simulink model "sampleModel2082"  (R2023a)
settings: Solver=VariableStepAuto  StartTime=0.0  StopTime=10.0  RelTol=1e-3
libraries: simulink x3, hdlsllib x2
settings Model: Creator=user1  LastModifiedBy=user1

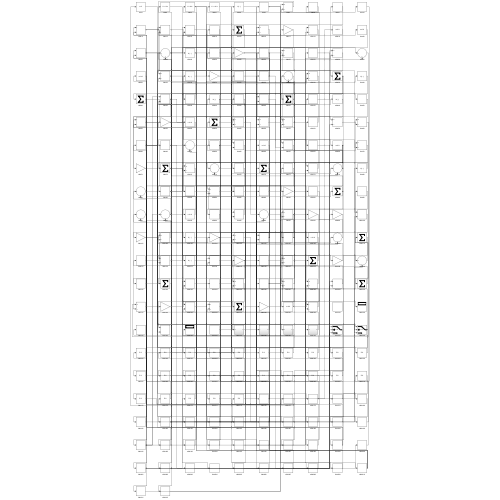
[thumbnail: Simulink's stored preview of the top-level diagram]
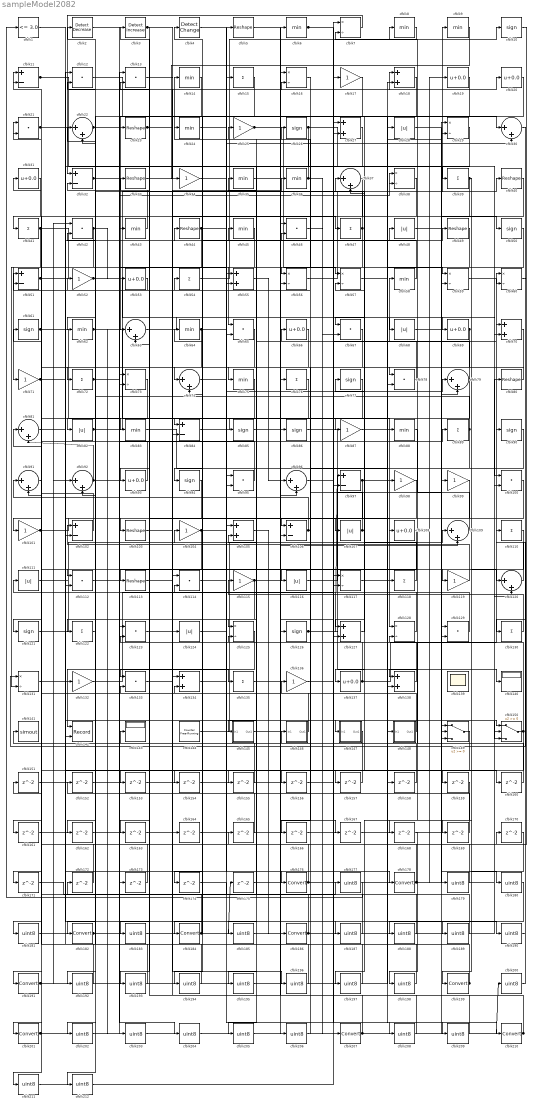
== system sampleModel2082 ==
  cfblk1 : hdlsllib/Logic and Bit Operations/Compare To Constant  relop=<=  const=3.0  OutDataTypeStr=boolean
  cfblk{10,26,50,61,77,85..86,90,94,121,126} (11 alike) : Signum
  cfblk{12..13,21,42,46,65,67,78,95,100,112,114,123,129,133} (15 alike) : DotProduct  OutDataTypeStr=Inherit: Inherit via internal rule
  cfblk{17,25,34,52,71,87,98..99,101,104,115,119,132,136} (14 alike) : Gain
  cfblk{11,32,51,84,97,102,106} (7 alike) : Sum  Inputs=+-
  cfblk{5,23,33,40,44,49,80,103,113} (9 alike) : Reshape
  cfblk{18,27,55,70,105,127,134,138} (8 alike) : Sum
  cfblk{28,48,68,82,107,111,116,124} (8 alike) : Abs  SaturateOnIntegerOverflow=off
  cfblk{19..20,31,53,66,69,93,108,137} (9 alike) : Bias  Bias=0.0  SaturateOnIntegerOverflow=off
  cfblk{22,30,37,63,74,79,81,91..92,96,109,120} (12 alike) : Sum  Inputs=|++
  cfblk{15,39,41,47,54,72,76,89,110,118,122,130,135} (13 alike) : Sum  Inputs=+
  cfblk{7,16,29,38,56..57,59..60,73,117,125,128,131} (13 alike) : Product  Inputs=*/  RndMeth=Zero  SaturateOnIntegerOverflow=on
  cfblk139 : Scope
      settings: Floating=on
  cfblk{6,8..9,14,24,35..36,43,45,58,62,64,75,83,88} (15 alike) : MinMax
  cfblk140 : Display
  cfblk141 : ToWorkspace  VariableName=simout  SaveFormat=Timeseries  SampleTime=-1
  cfblk142 : Record  FileSettingsInternal="{\"entries\":[{\"content\":{\"excelSettings\":{\"content\":{},\"type\":\"Streamout.ExcelSettings\"}},\"type\":\"Streamout.FileSettingStorage\",\"uuid\":\"\"}],\"packageUris\":[\"http:\\/\\/schema.mathworks.com\\/mf0\\/streamout_blocks\\/R2020a\"],\"version\":\"1.0\"}"  Layout=[1 1]  SignalsInternal="{\"entries\":[{\"content\":{\"signals\":[{\"content\":{\"blockPath\":[],\"dimensions\":[1],\"domain\":\"\",\"lineColor\":\"#a2142f\",\"plots\":[1],\"port\":1,\"signalID\":6656,\"signalName\":\"XY Graph:1\"},\"type\":\"RecordBlkView.Signal\",\"uuid\":\"\"},{\"content\":{\"blockPath\":[],\"dimensions\":[1],\"domain\":\"\",\"lineColor\":\"#139fff\",\"plots\":[1],\"port\":2,\"signalID\":6659,\"signalName\":\"XY Graph:2\"},\"type\":\"RecordBlkView.Signal\",\"uuid\":\"\"}]},\"type\":\"RecordBlkView.InputSignals\",\"uuid\":\"\"}],\"packageUris\":[\"http:\\/\\/schema.mathworks.com\\/mf0\\/streamout_blocks\\/R2020a\"],\"version\":\"1.0\"}"  VisualizationBindings="{\"xyplotplugin\":{\"info\":[{\"series\":[{\"bindingParametersList\":[{\"parameter\":\"X-Axis\",\"signalID\":6656,\"signalName\":\"XY Graph:1\"},{\"parameter\":\"Y-Axis\",\"signalID\":6659,\"signalName\":\"XY Graph:2\"}],\"seriesID\":13052}],\"subplotID\":1}]}}"  CompatibilityTag=XY  st=-1
  cfblk143 : Display
  cfblk144 : hdlsllib/Sources/Counter Free-Running  NumBits=16  tsamp=-1
  cfblk145 : Subsystem
      settings: LibrarySourceBlock=|
      | hdlsllib/Ports &
      | Subsystems/Subsystem
  cfblk146 : Subsystem
      settings: LibrarySourceBlock=|
      | hdlsllib/Ports &
      | Subsystems/Subsystem
  cfblk147 : Subsystem
      settings: LibrarySourceBlock=|
      | hdlsllib/Ports &
      | Subsystems/Subsystem
  cfblk148 : Subsystem
      settings: LibrarySourceBlock=|
      | hdlsllib/Ports &
      | Subsystems/Subsystem
  cfblk149 : Switch  SaturateOnIntegerOverflow=off  InputSameDT=off
  cfblk150 : Switch  SaturateOnIntegerOverflow=off  InputSameDT=off
  cfblk{151..175} (25 alike) : Delay  SampleTime=1
  cfblk{176,178,182,184,186,191,199,201,207,210} (10 alike) : DataTypeConversion  SaturateOnIntegerOverflow=off  RndMeth=Floor
  cfblk{177,179..181,183,185,187..190,192..198,200,202..206,208..209,211..212} (27 alike) : DataTypeConversion  OutDataTypeStr=uint8  SaturateOnIntegerOverflow=off  RndMeth=Floor
  cfblk2 : simulink/Logic and Bit Operations/Detect Decrease  vinit=0.0  OutDataTypeStr=boolean
      settings: LibrarySourceBlock=|
      | hdlsllib/Logic and Bit
      | Operations/Detect
      | Decrease
  cfblk3 : simulink/Logic and Bit Operations/Detect Increase  vinit=0.0  OutDataTypeStr=boolean
      settings: LibrarySourceBlock=|
      | hdlsllib/Logic and Bit
      | Operations/Detect
      | Increase
  cfblk4 : simulink/Logic and Bit Operations/Detect Change  vinit=0  OutDataTypeStr=boolean
      settings: LibrarySourceBlock=|
      | hdlsllib/Logic and Bit
      | Operations/Detect
      | Change
  wires:
  cfblk79/1 -> cfblk58/1, cfblk37/2, cfblk171/1
  cfblk101/1 -> cfblk103/1, cfblk150/2
  cfblk46/1 -> cfblk207/1
  cfblk31/1 -> cfblk41/1
  cfblk7/1 -> cfblk32/1
  cfblk86/1 -> cfblk140/1
  cfblk47/1 -> cfblk2/1, cfblk145/1(In1)
  cfblk55/1 -> cfblk96/1
  cfblk125/1 -> cfblk142/1
  cfblk84/1 -> cfblk87/1
  cfblk128/1 -> cfblk111/1
  cfblk82/1 -> cfblk40/1, cfblk38/2
  cfblk1/1 -> cfblk176/1
  cfblk36/1 -> cfblk14/1, cfblk67/2
  cfblk63/1 -> cfblk69/1
  cfblk91/1 -> cfblk191/1
  cfblk9/1 -> cfblk34/1
  cfblk45/1 -> cfblk71/1
  cfblk147/1(Out1) -> cfblk141/1
  cfblk3/1 -> cfblk43/1, cfblk47/1, cfblk187/1
  cfblk94/1 -> cfblk113/1
  cfblk54/1 -> cfblk10/1
  cfblk20/1 -> cfblk74/1
  cfblk121/1 -> cfblk104/1
  cfblk127/1 -> cfblk37/1
  cfblk61/1 -> cfblk83/1, cfblk44/1, cfblk108/1, cfblk155/1
  cfblk56/1 -> cfblk9/1
  cfblk129/1 -> cfblk35/1
  cfblk138/1 -> cfblk54/1
  cfblk30/1 -> cfblk131/1
  cfblk33/1 -> cfblk18/1
  cfblk148/1(Out1) -> cfblk64/1
  cfblk65/1 -> cfblk121/1
  cfblk34/1 -> cfblk95/1
  cfblk126/1 -> cfblk97/1, cfblk138/2
  cfblk44/1 -> cfblk133/1, cfblk156/1
  cfblk24/1 -> cfblk85/1
  cfblk62/1 -> cfblk128/1, cfblk203/1
  cfblk144/1 -> cfblk109/1
  cfblk25/1 -> cfblk57/1, cfblk127/2
  cfblk17/1 -> cfblk182/1
  cfblk75/1 -> cfblk93/1
  cfblk104/1 -> cfblk38/1, cfblk202/1
  cfblk117/1 -> cfblk210/1
  cfblk11/1 -> cfblk97/2, cfblk16/2
  cfblk102/1 -> cfblk21/1
  cfblk120/1 -> cfblk60/1
  cfblk41/1 -> cfblk49/1, cfblk131/2
  cfblk116/1 -> cfblk29/1
  cfblk32/1 -> cfblk122/1, cfblk150/1
  cfblk14/1 -> cfblk63/1
  cfblk150/1 -> cfblk33/1, cfblk163/1
  cfblk145/1(Out1) -> cfblk86/1
  cfblk50/1 -> cfblk65/1
  cfblk59/1 -> cfblk60/2
  cfblk21/1 -> cfblk39/1, cfblk190/1
  cfblk119/1 -> cfblk102/1
  cfblk90/1 -> cfblk106/1
  cfblk95/1 -> cfblk22/1
  cfblk132/1 -> cfblk7/1
  cfblk130/1 -> cfblk115/1
  cfblk103/1 -> cfblk116/1
  cfblk48/1 -> cfblk50/1
  cfblk112/1 -> cfblk89/1
  cfblk137/1 -> cfblk90/1, cfblk125/2
  cfblk23/1 -> cfblk70/2, cfblk193/1
  cfblk16/1 -> cfblk56/1
  cfblk76/1 -> cfblk184/1
  cfblk13/1 -> cfblk107/1
  cfblk52/1 -> cfblk124/1, cfblk20/1
  cfblk106/1 -> cfblk11/1, cfblk26/1
  cfblk43/1 -> cfblk32/2
  cfblk40/1 -> cfblk137/1
  cfblk8/1 -> cfblk7/2
  cfblk80/1 -> cfblk78/1
  cfblk29/1 -> cfblk142/2
  cfblk6/1 -> cfblk68/1, cfblk120/1
  cfblk5/1 -> cfblk126/1
  cfblk19/1 -> cfblk67/1
  cfblk146/1(Out1) -> cfblk51/1
  cfblk26/1 -> cfblk100/1, cfblk112/1, cfblk102/2
  cfblk42/1 -> cfblk53/1, cfblk181/1
  cfblk114/1 -> cfblk79/1
  cfblk4/1 -> cfblk178/1
  cfblk109/1 -> cfblk8/1
  cfblk69/1 -> cfblk84/1, cfblk84/2, cfblk157/1
  cfblk110/1 -> cfblk199/1
  cfblk53/1 -> cfblk51/2
  cfblk18/1 -> cfblk94/1
  cfblk73/1 -> cfblk82/1
  cfblk27/1 -> cfblk75/1
  cfblk133/1 -> cfblk36/1
  cfblk105/1 -> cfblk186/1
  cfblk64/1 -> cfblk30/2, cfblk153/1
  cfblk115/1 -> cfblk45/1, cfblk109/2, cfblk212/1
  cfblk111/1 -> cfblk27/2
  cfblk81/1 -> cfblk132/1
  cfblk83/1 -> cfblk148/1(In1)
  cfblk118/1 -> cfblk77/1
  cfblk67/1 -> cfblk72/1
  cfblk51/1 -> cfblk5/1, cfblk150/3
  cfblk38/1 -> cfblk62/1
  cfblk39/1 -> cfblk101/1, cfblk112/2, cfblk169/1
  cfblk97/1 -> cfblk29/2, cfblk125/1
  cfblk107/1 -> cfblk52/1, cfblk57/2, cfblk127/1
  cfblk49/1 -> cfblk73/2
  cfblk57/1 -> cfblk59/1
  cfblk72/1 -> cfblk135/1, cfblk204/1
  cfblk2/1 -> cfblk23/1
  cfblk71/1 -> cfblk147/1(In1), cfblk161/1
  cfblk124/1 -> cfblk15/1
  cfblk60/1 -> cfblk130/1
  cfblk93/1 -> cfblk61/1
  cfblk92/1 -> cfblk119/1, cfblk81/2
  cfblk78/1 -> cfblk25/1
  cfblk136/1 -> cfblk70/1
  cfblk22/1 -> cfblk55/2, cfblk30/1
  cfblk89/1 -> cfblk138/1, cfblk12/2
  cfblk12/1 -> cfblk88/1
  cfblk134/1 -> cfblk48/1
  cfblk149/1 -> cfblk201/1
  cfblk58/1 -> cfblk24/1
  cfblk151/1 -> cfblk73/1
  cfblk152/1 -> cfblk95/2
  cfblk153/1 -> cfblk106/2
  cfblk131/1 -> cfblk154/1
  cfblk154/1 -> cfblk55/1
  cfblk155/1 -> cfblk13/1
  cfblk156/1 -> cfblk27/1
  cfblk157/1 -> cfblk63/2
  cfblk87/1 -> cfblk158/1
  cfblk158/1 -> cfblk16/1
  cfblk135/1 -> cfblk159/1
  cfblk74/1 -> cfblk160/1
  cfblk160/1 -> cfblk128/2
  cfblk161/1 -> cfblk65/2
  cfblk122/1 -> cfblk162/1
  cfblk162/1 -> cfblk59/2
  cfblk163/1 -> cfblk96/2
  cfblk113/1 -> cfblk164/1
  cfblk164/1 -> cfblk18/2
  cfblk10/1 -> cfblk165/1
  cfblk165/1 -> cfblk22/2
  cfblk70/1 -> cfblk166/1
  cfblk166/1 -> cfblk78/2
  cfblk35/1 -> cfblk167/1
  cfblk167/1 -> cfblk79/2
  cfblk88/1 -> cfblk168/1
  cfblk169/1 -> cfblk133/2
  cfblk172/1 -> cfblk11/2
  cfblk173/1 -> cfblk42/2
  cfblk100/1 -> cfblk174/1
  cfblk175/1 -> cfblk56/2
  cfblk176/1 -> cfblk92/2, cfblk120/2, cfblk31/1
  cfblk171/1 -> cfblk177/1
  cfblk177/1 -> cfblk1/1
  cfblk178/1 -> cfblk134/2, cfblk19/1
  cfblk68/1 -> cfblk179/1
  cfblk179/1 -> cfblk4/1
  cfblk28/1 -> cfblk180/1
  cfblk181/1 -> cfblk28/1
  cfblk182/1 -> cfblk175/1, cfblk100/2, cfblk6/1
  cfblk77/1 -> cfblk183/1
  cfblk183/1 -> cfblk17/1
  cfblk184/1 -> cfblk81/1, cfblk80/1, cfblk74/2
  cfblk99/1 -> cfblk185/1
  cfblk185/1 -> cfblk76/1
  cfblk186/1 -> cfblk152/1, cfblk151/1, cfblk13/2
  cfblk187/1 -> cfblk105/1
  cfblk168/1 -> cfblk188/1
  cfblk188/1 -> cfblk105/2
  cfblk170/1 -> cfblk189/1
  cfblk189/1 -> cfblk114/2
  cfblk190/1 -> cfblk170/1
  cfblk191/1 -> cfblk118/1, cfblk92/1, cfblk42/1
  cfblk15/1 -> cfblk192/1
  cfblk192/1 -> cfblk91/1
  cfblk193/1 -> cfblk91/2
  cfblk98/1 -> cfblk194/1
  cfblk194/1 -> cfblk21/2
  cfblk37/1 -> cfblk195/1
  cfblk195/1 -> cfblk98/1
  cfblk123/1 -> cfblk196/1
  cfblk196/1 -> cfblk134/1
  cfblk159/1 -> cfblk197/1
  cfblk197/1 -> cfblk123/1
  cfblk180/1 -> cfblk198/1
  cfblk198/1 -> cfblk123/2
  cfblk199/1 -> cfblk172/1, cfblk12/1
  cfblk200/1 -> cfblk110/1
  cfblk201/1 -> cfblk200/1, cfblk173/1, cfblk99/1
  cfblk202/1 -> cfblk149/1
  cfblk203/1 -> cfblk149/2
  cfblk204/1 -> cfblk149/3
  cfblk66/1 -> cfblk205/1
  cfblk205/1 -> cfblk129/1
  cfblk85/1 -> cfblk206/1
  cfblk206/1 -> cfblk66/1
  cfblk207/1 -> cfblk129/2, cfblk3/1
  cfblk96/1 -> cfblk208/1
  cfblk208/1 -> cfblk46/1
  cfblk174/1 -> cfblk209/1
  cfblk209/1 -> cfblk46/2
  cfblk210/1 -> cfblk114/1, cfblk136/1, cfblk143/1, cfblk146/1(In1)
  cfblk108/1 -> cfblk211/1
  cfblk211/1 -> cfblk117/1
  cfblk212/1 -> cfblk117/2

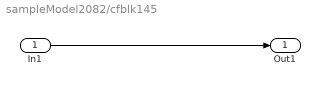
== system sampleModel2082/cfblk145 ==
  In1 : Inport
  Out1 : Outport
  wires:
  In1/1 -> Out1/1

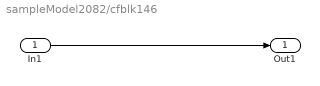
== system sampleModel2082/cfblk146 ==
  In1 : Inport
  Out1 : Outport
  wires:
  In1/1 -> Out1/1

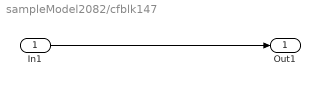
== system sampleModel2082/cfblk147 ==
  In1 : Inport
  Out1 : Outport
  wires:
  In1/1 -> Out1/1

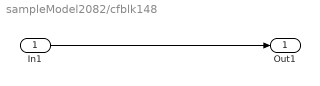
== system sampleModel2082/cfblk148 ==
  In1 : Inport
  Out1 : Outport
  wires:
  In1/1 -> Out1/1
